simulink model "PMSM_ClosedLoop_s32k144"  (Simulink 9.0)
settings: Solver=FixedStepDiscrete  StartTime=0.0  StopTime=10  RelTol=1e-3  EnableMultiTasking=on
model workspace (MAT data in the model file):
  C_LST = 0.0001
  FORCE_MODE_SPEED = 20
  IDC_OVERCURRENT = 5
  IQ_REF_MAX = 2.3
  IQ_REF_TRACKING = 2
  I_MAX = 31.25
  Nmax = 10000
  PP = 2
  PhA_Offset = 16.025
  PhB_Offset = 16.04
  SPEED_DOWN_INC = 5
  SPEED_LOOP_CNTR = 10
  SPEED_UP_INC = 5
  S_LST = 0.001
  TRACKING_MODE_SPEED = 40
  VDC_OVERVOLTAGE = 18
  VDC_UNDERVOLTAGE = 8
InitFcn:
  | mbd_s32k_consistency_checks(bdroot(gcs));
undefined symbols (not defined in the file): External, LQFP, One, Shot, TRGMUX_PDB_TRIG
libraries: mbd_s32k1xx_ec_toolbox x50, ammclib_bam_s32k14x x26, simulink x18, mbd_msd_ec_toolbox x5
(part 1 of 2)
Description:
  | Closed Loop Speed Control PMSM example for S32K144 and DevKit MotorGD.
  | This Simulink model is designed to work with Linix 45ZWN24-40 Motor and validate
  | that the motor can be based on FOC method.
  | 
  | FEATURES:
  | - Speed command is read via SW2 (CW direction) or SW3 (CCW direction)
  | - Motor starts by default in CW direction. Use SW3 to decrease speed and move CCW.
  |   Alternatively, use FreeMASTER pannel to control the speed and direction
  | - Measure the 3-phase sinusoidal currents with PWM-PDB-ADC synchronization
  | - Measure the DC bus voltage and current with PWM-PDB-ADC synchronization
  | - PI Speed, Flux and Torque Controllers
  | - Speed estimator based on HALL sensors
  | 
  | HW SETUP:
  | - Configure S32K144 board supply voltage: J107:2-3(over USB)
  | - Configure J9,J10 and J11 on MotorGD: 2-3 (mode BLDC)
  | - Rotate trimmer resistor R72 (placed Devkit-MotorGD) counter-clockwise at maximum
  | - Connect the motor phases to MotorGD J13 connector
  |   (i.e. Linix 45ZWN24-40: phA-white/phB-blue/phC-green)
  | - Connect the motor hall sensors to MotorGD JP1 connector
  |   (i.e. Linix 45ZWN24-40: Hall_A-white/Hall_B-blue/Hall_C-green)
  | - Power on the MotorGD via J7 connector with 12Vdc
  | - NOTE! Make sure the R168/R166 are placed and R167/R165 are removed.
  |             Required for speed estimator based on hall sensor
  | 
  | VALIDATION:
  | - After reset or power on, the Green LED shall be ON
  | - In case of a FAULT the Red LED will be ON
  | - The initial speed command is set to 500rpm and can be changed from Simulink Model Wrks
  | - Open FreeMASTER project and connect to the target.
  | - Start by pressing the SW2 or SW3 to command the motor to spin
  | - Press the SW2 or SW3 the modify the motor speed or use FreeMASTER UI panel
  | - Voltage and Current protections for Devkit MotorGD are enabled. If fault occurs the
  |   INVERTER is shut down and RED LED is ON
  | 
  | NOTE:
  | - In case of fault (RED LED is ON), the remove fault cause and press RESET button
  | 
  | Copyright (c) 2019 NXP
  | version 3.2.0
settings Model: SuppressorTable="22 serialization::archive 15 0 6 0 0 1 8 0 0 0 0 6 0 0 1 0 97 PMSM_ClosedLoop_s32k144/S32K144 EVB/IO Controls/Alignment/Repeating Sequence Stair/LimitedCounter 0 6 0 0 2 8 0 0 0 0 6 40 SimulinkFixedPoint:util:Overflowoccurred 0 0 0 6 0  0  0 0 0 0 8 20160608 0 0 0 15 23 17 0 1 41 Simulink:DataType:WarningOverFlowDetected 0 0 0  0  8 20160608 0 15 23 17 0 1"  Creator=NXP MBDT Team  LastModifiedBy=nxf40284  OrderedModelArguments=off
settings DataIOCC: ExternalInput=off  InitialState=off  LimitDataPoints=on  SaveOutput=off  SignalLogging=off  SaveTime=off
settings OptimizationCC: DefaultParameterBehavior=Inlined  UseFloatMulNetSlope=on  DefaultUnderspecifiedDataType=single  UseSpecifiedMinMax=on  EnhancedBackFolding=on  PassReuseOutputArgsAs=Individual arguments  ZeroExternalMemoryAtStartup=off  ZeroInternalMemoryAtStartup=off  NoFixptDivByZeroProtection=on  EfficientFloat2IntCast=on  LifeSpan=auto  OptimizeBlockOrder=speed  DifferentSizesBufferReuse=on
settings DebuggingCC: CheckSSInitialOutputMsg=off  SolverPrmCheckMsg=warning  InheritedTsInSrcMsg=none  MultiTaskDSMMsg=none  SingleTaskRateTransMsg=error  ParameterPrecisionLossMsg=none  ParameterTunabilityLossMsg=error  UnconnectedInputMsg=error  UnconnectedOutputMsg=error  UnconnectedLineMsg=error  AssertControl=DisableAll  AllowSymbolicDim=off  UnknownTsInhSupMsg=error  StateNameClashWarn=warning  SFSelfTransitionDiag=none
settings HardwareCC: ProdLargestAtomicInteger=Long  ProdLargestAtomicFloat=Double  ProdIntDivRoundTo=Zero  ProdEndianess=LittleEndian  ProdHWDeviceType=ARM Compatible->ARM Cortex
settings ModelReferenceCC: PropagateSignalLabelsOutOfModel=on
settings SFSimCC: MATLABDynamicMemAlloc=off
settings RTWCC: SystemTargetFile=mbd_s32k.tlc  MakeCommand=mbd_s32k_make_rtw COPY_MDLREF_INCLUDES=0  TemplateMakefile=mbd_s32k.tmf  Description=Model Based Design Toolbox S32K1xx Code Generation Target  IncludeHyperlinkInReport=on
settings CodeAppCC: ForceParamTrailComments=on  IgnoreCustomStorageClasses=off  MaxIdLength=64  OperatorAnnotations=on  SimulinkDataObjDesc=on  SFDataObjDesc=on  InsertBlockDesc=on  StateflowObjectComments=off  InternalIdentifier=Classic
settings STFCustomTargetCC: TargetLangStandard=C99 (ISO)  MultiwordLength=256  CombineOutputUpdateFcns=on  ERTCustomFileBanners=on  SupportContinuousTime=off  SupportNonInlinedSFcns=off  RemoveResetFunc=on  MATLABClassNameForMDSCustomization=Simulink.SoftwareTarget.ERTCustomization  GRTInterface=off  SystemTargetFile=mbd_s32k.tlc
settings ERTTargetCC: TargetLangStandard=C99 (ISO)  ParMdlRefBuildCompliant=off  CompOptLevelCompliant=off  ConcurrentExecutionCompliant=off  ModelStepFunctionPrototypeControlCompliant=off  CPPClassGenCompliant=off  UseToolchainInfoCompliant=off  InlinedParameterPlacement=NonHierarchical  ERTSrcFileBannerTemplate=mbd_ert_code_template.cgt  ERTHdrFileBannerTemplate=mbd_ert_code_template.cgt  ERTDataSrcFileTemplate=mbd_ert_code_template.cgt  ERTDataHdrFileTemplate=mbd_ert_code_template.cgt  ERTCustomFileTemplate=example_file_process.tlc

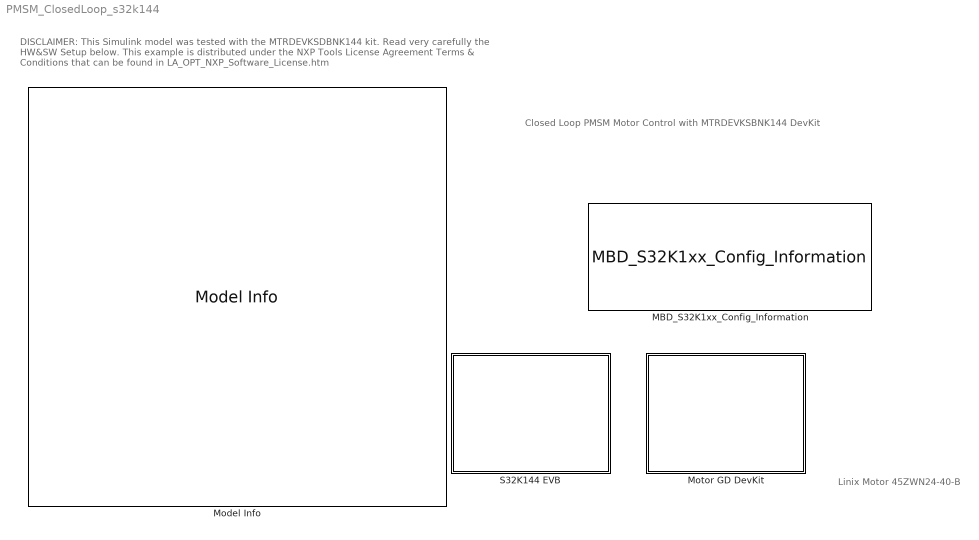
== system PMSM_ClosedLoop_s32k144 ==
  note: Linix Motor 45ZWN24-40-B
  note: Closed Loop PMSM Motor Control
      | with MTRDEVKSBNK144 DevKit
  note: DISCLAIMER: This Simulink model was tested with the MTRDEVKSDBNK144 kit. Read very carefully the HW&SW Setup below.
      | This example is distributed under the NXP Tools License Agreement Terms & Conditions that can be found in LA_OPT_NXP_Software_License.htm
  MBD_S32K1xx_Config_Information : mbd_s32k1xx_ec_toolbox/MBD_S32K1xx_Config_Information  mbdt_ver=0  disp_str=|  config_params=[]  mcu_target_name=S32K144  mcu_target_package=64-LQFP  mcu_target_sram_size=64KB  mcu_system_clock_freq=80  mcu_xtal_freq=External 8  mcu_steptick_timer=LPIT Channel 0  mcu_steptick_prio=15  ds_import_enable=on  target_compiler=GCC  target_memory=FLASH  gcc_target_compile_opts=-mcpu=cortex-m4 -mthumb -mfloat-abi=hard -mfpu=fpv4-sp-d16 -O1 -g -gstrict-dwarf  gcc_target_assemble_opts=-mcpu=cortex-m4 -mthumb -mfloat-abi=hard -mfpu=fpv4-sp-d16 -g  gcc_target_link_opts=-mcpu=cortex-m4 -mthumb -mfloat-abi=hard -mfpu=fpv4-sp-d16  gcc_target_default_lcf=on  gcc_target_user_lcf=S32K144_64_flash.ld  ghs_target_compile_opts=-cpu=cortexm4f -thumb -fpu=vfpv4_d16 -fsingle -Ogeneral -Wundef -Wimplicit-int -Wshadow -Wtrigraphs --no_commons --gnu_asm -gnu99 -gdwarf-2 -G  ghs_target_assemble_opts=-cpu=cortexm4f -fpu=vfpv4_d16  ghs_target_link_opts=-cpu=cortexm4f -thumb -fpu=vfpv4_d16  ghs_target_default_lcf=on  ghs_target_user_lcf=S32K144_64_flash.ld  iar_target_compile_opts=--cpu=Cortex-M4F --thumb --fpu=VFPv4_sp -Ol -e --debug --dlib_config normal  iar_target_assemble_opts=--cpu Cortex-M4F --thumb --fpu VFPv4_sp  iar_target_link_opts=--no_exceptions --vfe --inline  iar_target_default_lcf=on  iar_target_user_lcf=S32K144_64_flash.icf  pil_download_enable=off  rbl_download_enable=on  rbl_start_delay=5000  rbl_download_interface=OpenSDA  rbl_restart_request=off  rbl_com_port=Custom  rbl_com_port_custom=COM1  pil_download_rate=57600  pil_opensda_drive=Custom  pil_opensda_drive_custom=D  pil_uart_instance=1  pil_uart_rx=PTC6: [LPUART1_RX | Receive]  pil_uart_tx=PTC7: [LPUART1_TX | Transmit]  FTM_PWM_PcrCheckEnDis=on  FTM_Input_Edge_Inputs_PcrCheckEnDis=on  FTM_Dual_Edge_Inputs_PcrCheckEnDis=on  FTM_Quadrature_Inputs_PcrCheckEnDis=on  FTM_Hall_Sensor_Inputs_PcrCheckEnDis=on  LPTMR_PcrCheckEnDis=on  PIT_PcrCheckEnDis=on  RTC_PcrCheckEnDis=on  FlexCAN_PcrCheckEnDis=on  LIN_PcrCheckEnDis=on  FlexIO_PcrCheckEnDis=on  LPI2C_PcrCheckEnDis=on  LPSPI_PcrCheckEnDis=on  LPUART_PcrCheckEnDis=on  CMP_PcrCheckEnDis=on  GPIO_OutputPcrCheckEnDis=on  GPIO_InputPcrCheckEnDis=on  SBC_PcrCheckEnDis=on  AMMCLIB_PcrCheckEnDis=on  FM_PcrCheckEnDis=on  Profile_PcrCheckEnDis=on  ConfigParams_PcrCheckEnDis=on  ModelRef_PcrCheckEnDis=on  PDB0_PcrCheckEnDis=on  CSEc_PcrCheckEnDis=on  eDMA_PcrCheckEnDis=on  ADC_PcrCheckEnDis=on  WDOG_PcrCheckEnDis=on
      | Target : S32K144-64KB_SRAM
      | Package : 100-pin
      | System clock : 80 MHz
      | XTAL clock : External 8 MHz
      | Compiler : IAR
      | Target Type : FLASH
      | Download Code after build : off
      | Step Tick Interrupt Priority : 15
  Model Info : simulink/Model-Wide Utilities/Model Info  Frame=off  DisplayStringWithTags=|  HorizontalTextAlignment=Left  LeftAlignmentValue=0.02
      | Model Name: %<ModelName>
      | 
      | Description: %<Description>
  Motor GD DevKit : Subsystem
      mask Display: image('MotorGD.PNG');
  S32K144 EVB : Subsystem
      mask Display: image('S32K.PNG');

== system PMSM_ClosedLoop_s32k144/Motor GD DevKit ==

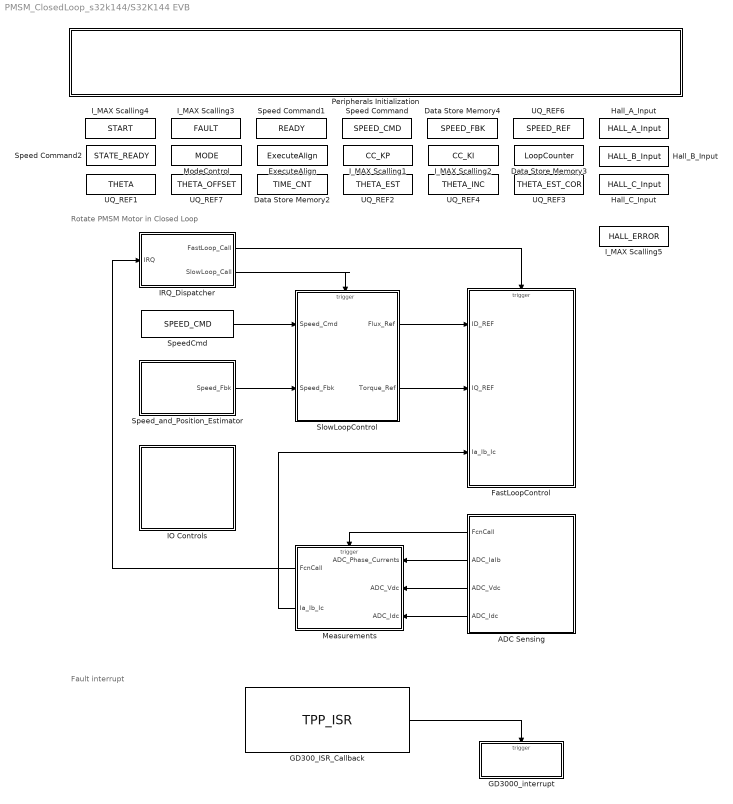
== system PMSM_ClosedLoop_s32k144/S32K144 EVB ==
  note: Rotate PMSM Motor in Closed Loop
  note: Fault interrupt
  ADC Sensing : Subsystem
  Data Store Memory2 : DataStoreMemory  DataStoreName=TIME_CNT  ReadBeforeWriteMsg=warning  WriteAfterWriteMsg=warning  WriteAfterReadMsg=warning  ShowAdditionalParam=off  OutDataTypeStr=uint32
  Data Store Memory3 : DataStoreMemory  DataStoreName=LoopCounter  ReadBeforeWriteMsg=warning  WriteAfterWriteMsg=warning  WriteAfterReadMsg=warning  ShowAdditionalParam=off  OutDataTypeStr=uint16
  Data Store Memory4 : DataStoreMemory  DataStoreName=SPEED_FBK  ReadBeforeWriteMsg=warning  WriteAfterWriteMsg=warning  WriteAfterReadMsg=warning  ShowAdditionalParam=off  OutDataTypeStr=single
      settings: RTWStateStorageClass=ExportedGlobal
  ExecuteAlign : DataStoreMemory  DataStoreName=ExecuteAlign  ReadBeforeWriteMsg=warning  WriteAfterWriteMsg=warning  WriteAfterReadMsg=warning  ShowAdditionalParam=off  OutDataTypeStr=boolean
      settings: RTWStateStorageClass=ExportedGlobal
  FastLoopControl : Subsystem
      settings: RTWSystemCode=Nonreusable function  RTWFcnNameOpts=Use subsystem name
  GD3000_interrupt : Subsystem  TreatAsAtomicUnit=on
  "GD300_ISR_Callback " : mbd_msd_ec_toolbox/TPP/TPP_ISR  tppInstance=0
  Hall_A_Input : DataStoreMemory  DataStoreName=HALL_A_Input  ReadBeforeWriteMsg=warning  WriteAfterWriteMsg=warning  WriteAfterReadMsg=warning  ShowAdditionalParam=off  OutDataTypeStr=boolean
  Hall_B_Input : DataStoreMemory  DataStoreName=HALL_B_Input  ReadBeforeWriteMsg=warning  WriteAfterWriteMsg=warning  WriteAfterReadMsg=warning  ShowAdditionalParam=off  OutDataTypeStr=boolean
  Hall_C_Input : DataStoreMemory  DataStoreName=HALL_C_Input  ReadBeforeWriteMsg=warning  WriteAfterWriteMsg=warning  WriteAfterReadMsg=warning  ShowAdditionalParam=off  OutDataTypeStr=boolean
  IO Controls : Subsystem
  IRQ_Dispatcher : Subsystem
      settings: MinAlgLoopOccurrences=on
  I_MAX Scalling1 : DataStoreMemory  DataStoreName=CC_KP  ReadBeforeWriteMsg=warning  WriteAfterWriteMsg=warning  WriteAfterReadMsg=warning  InitialValue=0.2  ShowAdditionalParam=off  OutDataTypeStr=single
  I_MAX Scalling2 : DataStoreMemory  DataStoreName=CC_KI  ReadBeforeWriteMsg=warning  WriteAfterWriteMsg=warning  WriteAfterReadMsg=warning  InitialValue=0.25  ShowAdditionalParam=off  OutDataTypeStr=single
  I_MAX Scalling3 : DataStoreMemory  DataStoreName=FAULT  ReadBeforeWriteMsg=warning  WriteAfterWriteMsg=warning  WriteAfterReadMsg=warning  ShowAdditionalParam=off  OutDataTypeStr=boolean
  I_MAX Scalling4 : DataStoreMemory  DataStoreName=START  ReadBeforeWriteMsg=warning  WriteAfterWriteMsg=warning  WriteAfterReadMsg=warning  ShowAdditionalParam=off  OutDataTypeStr=boolean
  I_MAX Scalling5 : DataStoreMemory  DataStoreName=HALL_ERROR  ReadBeforeWriteMsg=warning  WriteAfterWriteMsg=warning  WriteAfterReadMsg=warning  ShowAdditionalParam=off  OutDataTypeStr=uint8
  Measurements : Subsystem  TreatAsAtomicUnit=on
  ModeControl : DataStoreMemory  DataStoreName=MODE  ReadBeforeWriteMsg=warning  WriteAfterWriteMsg=warning  WriteAfterReadMsg=warning  ShowAdditionalParam=off  OutMin=0  OutMax=2  OutDataTypeStr=uint16
      settings: RTWStateStorageClass=ExportedGlobal
  Peripherals Initialization : Subsystem  Priority=1
  SlowLoopControl : Subsystem
      settings: PropExecContextOutsideSubsystem=on  RTWSystemCode=Nonreusable function  RTWFcnNameOpts=Use subsystem name
  Speed Command : DataStoreMemory  DataStoreName=SPEED_CMD  ReadBeforeWriteMsg=warning  WriteAfterWriteMsg=warning  WriteAfterReadMsg=warning  InitialValue=52.35  ShowAdditionalParam=off  OutMin=0  OutMax=209.4  OutDataTypeStr=single
  Speed Command1 : DataStoreMemory  DataStoreName=READY  ReadBeforeWriteMsg=warning  WriteAfterWriteMsg=warning  WriteAfterReadMsg=warning  ShowAdditionalParam=off  OutMin=0  OutMax=1  OutDataTypeStr=boolean
  Speed Command2 : DataStoreMemory  DataStoreName=STATE_READY  ReadBeforeWriteMsg=warning  WriteAfterWriteMsg=warning  WriteAfterReadMsg=warning  ShowAdditionalParam=off  OutMin=0  OutMax=1  OutDataTypeStr=boolean
  SpeedCmd : DataStoreRead  DataStoreName=SPEED_CMD
  Speed_and_Position_Estimator : Subsystem  TreatAsAtomicUnit=on
      settings: RTWFcnNameOpts=Use subsystem name
  UQ_REF1 : DataStoreMemory  DataStoreName=THETA  ReadBeforeWriteMsg=warning  WriteAfterWriteMsg=warning  WriteAfterReadMsg=warning  ShowAdditionalParam=off  OutDataTypeStr=single
  UQ_REF2 : DataStoreMemory  DataStoreName=THETA_EST  ReadBeforeWriteMsg=warning  WriteAfterWriteMsg=warning  WriteAfterReadMsg=warning  ShowAdditionalParam=off  OutDataTypeStr=single
  UQ_REF3 : DataStoreMemory  DataStoreName=THETA_EST_COR  ReadBeforeWriteMsg=warning  WriteAfterWriteMsg=warning  WriteAfterReadMsg=warning  ShowAdditionalParam=off  OutDataTypeStr=single
  UQ_REF4 : DataStoreMemory  DataStoreName=THETA_INC  ReadBeforeWriteMsg=warning  WriteAfterWriteMsg=warning  WriteAfterReadMsg=warning  ShowAdditionalParam=off  OutDataTypeStr=single
  UQ_REF6 : DataStoreMemory  DataStoreName=SPEED_REF  ReadBeforeWriteMsg=warning  WriteAfterWriteMsg=warning  WriteAfterReadMsg=warning  ShowAdditionalParam=off  OutDataTypeStr=single
  UQ_REF7 : DataStoreMemory  DataStoreName=THETA_OFFSET  ReadBeforeWriteMsg=warning  WriteAfterWriteMsg=warning  WriteAfterReadMsg=warning  ShowAdditionalParam=off  OutDataTypeStr=single
  wires:
  Measurements/2(Ia_Ib_Ic) -> FastLoopControl/3(Ia_Ib_Ic)
  ADC Sensing/2(ADC_IaIb) -> Measurements/1(ADC_Phase_Currents)
  SlowLoopControl/2(Torque_Ref) -> FastLoopControl/2(IQ_REF)
  Measurements/1(FcnCall) -> IRQ_Dispatcher/1(IRQ)
  ADC Sensing/1(FcnCall) -> Measurements/Trigger
  ADC Sensing/3(ADC_Vdc) -> Measurements/2(ADC_Vdc)
  SlowLoopControl/1(Flux_Ref) -> FastLoopControl/1(ID_REF)
  IRQ_Dispatcher/2(SlowLoop_Call) -> SlowLoopControl/Trigger
  ADC Sensing/4(ADC_Idc) -> Measurements/3(ADC_Idc)
  IRQ_Dispatcher/1(FastLoop_Call) -> FastLoopControl/Trigger
  SpeedCmd/1 -> SlowLoopControl/1(Speed_Cmd)
  Speed_and_Position_Estimator/1(Speed_Fbk) -> SlowLoopControl/2(Speed_Fbk)
  "GD300_ISR_Callback "/1 -> GD3000_interrupt/Trigger

== system PMSM_ClosedLoop_s32k144/S32K144 EVB/ADC Sensing ==
  ADC1_IRQHandler : Subsystem  TreatAsAtomicUnit=on
  ADC1_ISR : mbd_s32k1xx_ec_toolbox/Motor Control Blocks/ADC Blocks/ADC_ISR  instance=1  pri=1  sc1n=C
  PDB1_IRQHandler : Subsystem  TreatAsAtomicUnit=on
  PDB1_ISR : mbd_s32k1xx_ec_toolbox/Motor Control Blocks/PDB Blocks/PDB_ISR  Priority=8  pdbModule=1  prioInterrupt=2  regScPdbie=on  regScPdbeie=off  regIdlyIdly=4999
  Terminator{,1..2,6} (4 alike) : Terminator
  FcnCall : Outport
  ADC_IaIb : Outport  Port=2
  ADC_Vdc : Outport  Port=3
  ADC_Idc : Outport  Port=4
  wires:
  PDB1_ISR/2 -> Terminator1/1
  PDB1_ISR/3 -> Terminator2/1
  PDB1_ISR/4 -> Terminator/1
  PDB1_ISR/1 -> PDB1_IRQHandler/Trigger
  ADC1_IRQHandler/3(ADC_Vdc) -> ADC_Vdc/1
  ADC1_IRQHandler/2(ADC_Phase_Currents) -> ADC_IaIb/1
  ADC1_IRQHandler/4(ADC_Idc) -> ADC_Idc/1
  ADC1_IRQHandler/1(FcnCall) -> FcnCall/1
  ADC1_ISR/1 -> ADC1_IRQHandler/Trigger
  ADC1_ISR/2 -> ADC1_IRQHandler/1(ADC_IB)
  ADC1_ISR/3 -> Terminator6/1

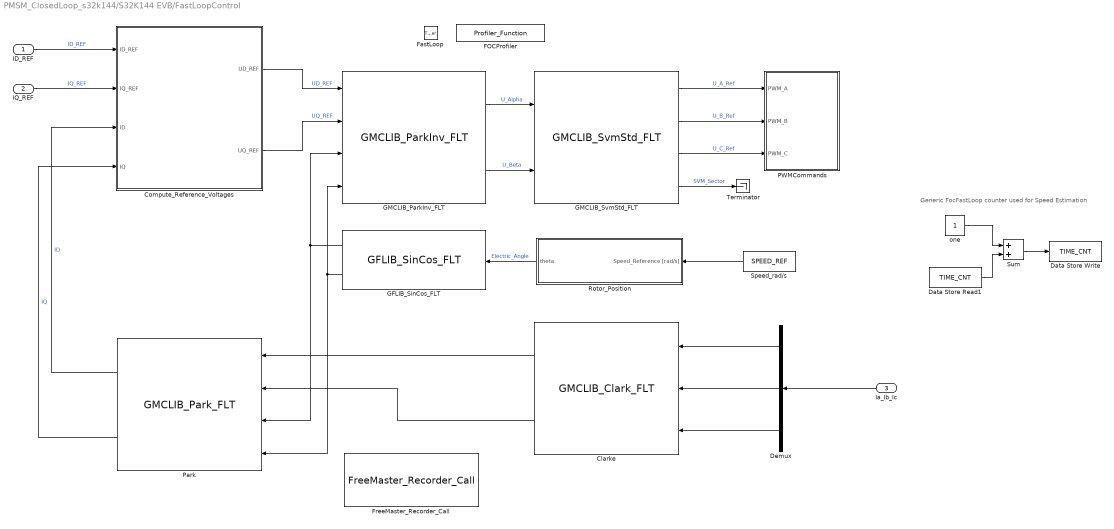
== system PMSM_ClosedLoop_s32k144/S32K144 EVB/FastLoopControl ==
  note: Generic FocFastLoop counter used for Speed Estimation
  ID_REF : Inport
  IQ_REF : Inport  Port=2
  Ia_Ib_Ic : Inport  Port=3
  FastLoop : TriggerPort  TriggerType=function-call  VariantControl=(inherit)
  Clarke : ammclib_bam_s32k14x/GMCLIB/bam_flt/GMCLIB_Clark_FLT
  Compute_Reference_Voltages : Subsystem
  Data Store Read1 : DataStoreRead  DataStoreName=TIME_CNT
  Data Store Write : DataStoreWrite  DataStoreName=TIME_CNT
  Demux : Demux  Outputs=3
  FOCProfiler : mbd_s32k1xx_ec_toolbox/Utility Blocks/Profiler_Function  profile_indx=2
  FreeMaster_Recorder_Call : mbd_s32k1xx_ec_toolbox/Utility Blocks/FreeMaster_Recorder_Call
  GFLIB_SinCos_FLT : ammclib_bam_s32k14x/GFLIB/bam_flt/GFLIB_SinCos_FLT
  GMCLIB_ParkInv_FLT : ammclib_bam_s32k14x/GMCLIB/bam_flt/GMCLIB_ParkInv_FLT
  GMCLIB_SvmStd_FLT : ammclib_bam_s32k14x/GMCLIB/bam_flt/GMCLIB_SvmStd_FLT
  PWMCommands : Subsystem
  Park : ammclib_bam_s32k14x/GMCLIB/bam_flt/GMCLIB_Park_FLT
  Rotor_Position : Subsystem
  Speed_rad/s : DataStoreRead  DataStoreName=SPEED_REF
  Sum : Sum
  Terminator : Terminator
  one : Constant  OutDataTypeStr=uint32
  wires:
  GFLIB_SinCos_FLT/2 -> Park/4, GMCLIB_ParkInv_FLT/4
  GMCLIB_ParkInv_FLT/1 -> GMCLIB_SvmStd_FLT/1  "U_Alpha"
  GMCLIB_ParkInv_FLT/2 -> GMCLIB_SvmStd_FLT/2  "U_Beta"
  GFLIB_SinCos_FLT/1 -> Park/3, GMCLIB_ParkInv_FLT/3
  GMCLIB_SvmStd_FLT/2 -> PWMCommands/2(PWM_B)  "U_B_Ref"
  GMCLIB_SvmStd_FLT/3 -> PWMCommands/3(PWM_C)  "U_C_Ref"
  GMCLIB_SvmStd_FLT/4 -> Terminator/1  "SVM_Sector"
  GMCLIB_SvmStd_FLT/1 -> PWMCommands/1(PWM_A)  "U_A_Ref"
  Compute_Reference_Voltages/1(UD_REF) -> GMCLIB_ParkInv_FLT/1  "UD_REF"
  Compute_Reference_Voltages/2(UQ_REF) -> GMCLIB_ParkInv_FLT/2  "UQ_REF"
  Rotor_Position/1(theta) -> GFLIB_SinCos_FLT/1  "Electric_Angle"
  Park/1 -> Compute_Reference_Voltages/3(ID)  "ID"
  IQ_REF/1 -> Compute_Reference_Voltages/2(IQ_REF)  "IQ_REF"
  Park/2 -> Compute_Reference_Voltages/4(IQ)  "IQ"
  ID_REF/1 -> Compute_Reference_Voltages/1(ID_REF)  "ID_REF"
  Demux/2 -> Clarke/2
  Demux/3 -> Clarke/3
  Ia_Ib_Ic/1 -> Demux/1
  Clarke/1 -> Park/1
  Clarke/2 -> Park/2
  Demux/1 -> Clarke/1
  one/1 -> Sum/1
  Data Store Read1/1 -> Sum/2
  Speed_rad/s/1 -> Rotor_Position/1(Speed_Reference [rad/s])
  Sum/1 -> Data Store Write/1

== system PMSM_ClosedLoop_s32k144/S32K144 EVB/GD3000_interrupt ==
  function : TriggerPort  TriggerType=function-call  VariantControl=Variant
  FAULT_write : DataStoreWrite  DataStoreName=FAULT
  FTM_PWM_Disable_Enable : mbd_s32k1xx_ec_toolbox/Motor Control Blocks/FTM Blocks/FTM_PWM_Disable_Enable  ftmModule=3  action=Disable
  NOK : Constant  OutDataTypeStr=boolean
  TPP_Functional_Mode : mbd_msd_ec_toolbox/TPP/TPP_Functional_Mode  tppInstance=0  action=Sleep
  wires:
  NOK/1 -> FAULT_write/1

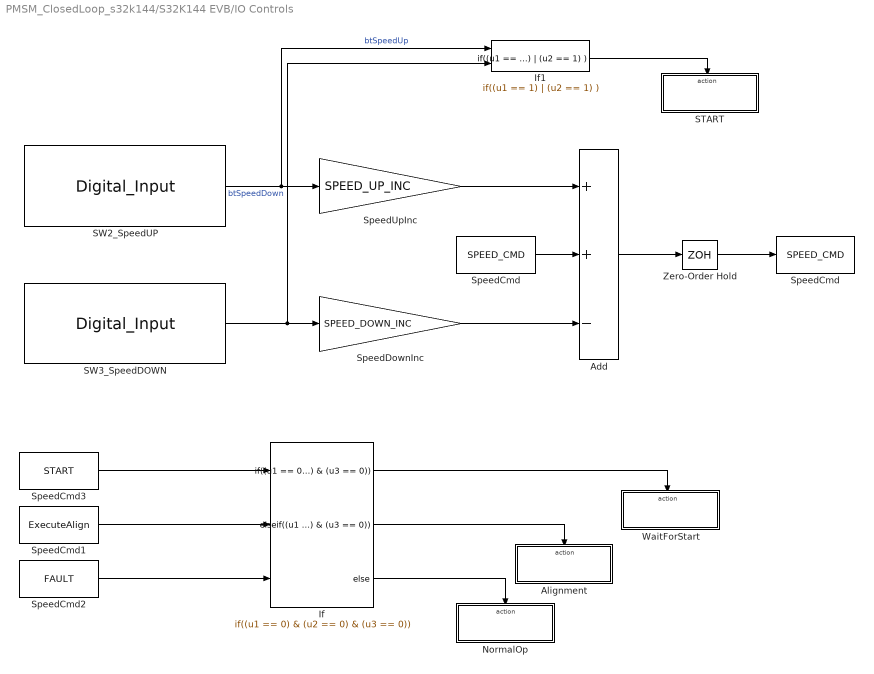
== system PMSM_ClosedLoop_s32k144/S32K144 EVB/IO Controls ==
  Add : Sum  Inputs=++-
  Alignment : Subsystem  TreatAsAtomicUnit=on
  If : If  NumInputs=3  IfExpression=(u1 == 0) & (u2 == 0) & (u3 == 0)  ElseIfExpressions=(u1 == 1) & (u2 ~= 0) & (u3 == 0)
  If1 : If  NumInputs=2  IfExpression=(u1 == 1) | (u2 == 1)  ShowElse=off
  NormalOp : Subsystem  TreatAsAtomicUnit=on
  START : Subsystem  TreatAsAtomicUnit=on
  SW2_SpeedUP : mbd_s32k1xx_ec_toolbox/GPIO Blocks/Digital_Input  gpio_pin=PTC12: [PTC12 | Port C I/O]  pull_resistor=None  passive_filter=off
  SW3_SpeedDOWN : mbd_s32k1xx_ec_toolbox/GPIO Blocks/Digital_Input  gpio_pin=PTC13: [PTC13 | Port C I/O]  pull_resistor=None  passive_filter=off
  SpeedCmd : DataStoreRead  DataStoreName=SPEED_CMD
  "SpeedCmd " : DataStoreWrite  DataStoreName=SPEED_CMD
  SpeedCmd1 : DataStoreRead  DataStoreName=ExecuteAlign
  SpeedCmd2 : DataStoreRead  DataStoreName=FAULT
  SpeedCmd3 : DataStoreRead  DataStoreName=START
  SpeedDownInc : Gain  Gain=SPEED_DOWN_INC  OutDataTypeStr=single
  SpeedUpInc : Gain  Gain=SPEED_UP_INC  OutDataTypeStr=single
  WaitForStart : Subsystem  TreatAsAtomicUnit=on
  Zero-Order Hold : ZeroOrderHold  SampleTime=0.25
  wires:
  Add/1 -> Zero-Order Hold/1
  SW3_SpeedDOWN/1 -> If1/2, SpeedDownInc/1  "btSpeedDown"
  SW2_SpeedUP/1 -> If1/1, SpeedUpInc/1  "btSpeedUp"
  SpeedCmd/1 -> Add/2
  SpeedUpInc/1 -> Add/1
  SpeedDownInc/1 -> Add/3
  Zero-Order Hold/1 -> "SpeedCmd "/1
  If1/1 -> START/Action
  SpeedCmd2/1 -> If/3
  SpeedCmd3/1 -> If/1
  If/1 -> WaitForStart/Action
  If/3 -> NormalOp/Action
  SpeedCmd1/1 -> If/2
  If/2 -> Alignment/Action

== system PMSM_ClosedLoop_s32k144/S32K144 EVB/IRQ_Dispatcher ==
  IRQ : Inport
  " " : DataStoreRead  DataStoreName=READY
  "  " : DataStoreRead  DataStoreName=START
  Generate_Triggers : Subsystem  TreatAsAtomicUnit=on
  Generate_Triggers_on_Startup : If  NumInputs=2  IfExpression=(u1 == 0) & (u2 == 1)  ShowElse=off
  Mux1 : Mux  Inputs=2
  Trigger_FastLoop_Call : Subsystem  TreatAsAtomicUnit=on
  FastLoop_Call : Outport
  SlowLoop_Call : Outport  Port=2
  wires:
  " "/1 -> Generate_Triggers_on_Startup/1
  Generate_Triggers_on_Startup/1 -> Trigger_FastLoop_Call/Action
  Trigger_FastLoop_Call/1(Call) -> Mux1/1
  Mux1/1 -> FastLoop_Call/1
  IRQ/1 -> Generate_Triggers/Trigger
  Generate_Triggers/1(FastLoop_Call) -> Mux1/2
  Generate_Triggers/2(SlowLoop_Call) -> SlowLoop_Call/1
  "  "/1 -> Generate_Triggers_on_Startup/2

== system PMSM_ClosedLoop_s32k144/S32K144 EVB/Measurements ==
  ADC_Phase_Currents : Inport
  ADC_Vdc : Inport  Port=2
  ADC_Idc : Inport  Port=3
  function : TriggerPort  TriggerType=function-call  VariantControl=(inherit)
  FaultDetection : Subsystem  TreatAsAtomicUnit=on
  Function-Call Generator : simulink/Ports & Subsystems/Function-Call Generator  Priority=4  sample_time=-1  numberOfIterations=1
  Get3PhCurrent : Subsystem  Priority=1  TreatAsAtomicUnit=on
  GetIdcCurrent : Subsystem  Priority=3  TreatAsAtomicUnit=on
      settings: RTWFcnNameOpts=Use subsystem name
  GetVdcVoltage : Subsystem  Priority=2  TreatAsAtomicUnit=on
      settings: RTWFcnNameOpts=Use subsystem name
  FcnCall : Outport
  Ia_Ib_Ic : Outport  Port=2
  wires:
  ADC_Vdc/1 -> GetVdcVoltage/1(ADC_Vdc)
  GetIdcCurrent/1(Idc) -> FaultDetection/2(Idc)
  GetVdcVoltage/1(Vdc) -> FaultDetection/1(Vdc)
  ADC_Phase_Currents/1 -> Get3PhCurrent/1(ADC_Phase_Currents)
  ADC_Idc/1 -> GetIdcCurrent/1(ADC_Idc)
  Get3PhCurrent/1(Ia_Ib_Ic) -> Ia_Ib_Ic/1
  Function-Call Generator/1 -> FcnCall/1

== system PMSM_ClosedLoop_s32k144/S32K144 EVB/Peripherals Initialization ==
  ADC0_Init : mbd_s32k1xx_ec_toolbox/Motor Control Blocks/ADC Blocks/ADC_Config  Priority=3  instance=0  mode=12-bit conversion  smplts=2  adiclk=alternate clock 1  adiv=input clock  show_adv_opts=on  pretrgsel=PDB pre-trigger  swpretrg=Disabled  adtrg=hardware  trgsel=PDB output  refsel=Vrefh and Vrefl  supply_monitoring=off  acfe=off  acfgt=off  acren=off  cv1=0  cv2=0  adco=off  avge=off  avgs=4 samples
  ADC1_IRQ : mbd_s32k1xx_ec_toolbox/Motor Control Blocks/ADC Blocks/ADC_Start  Priority=5  instance=1  adc_r=C  adc_chan=PTB16: [ADC1_SE15 | ADC Single Ended Input]  aien=on  mcuTargetUpdate=on
  ADC1_Init : mbd_s32k1xx_ec_toolbox/Motor Control Blocks/ADC Blocks/ADC_Config  Priority=4  instance=1  mode=12-bit conversion  smplts=2  adiclk=alternate clock 1  adiv=input clock  show_adv_opts=on  pretrgsel=PDB pre-trigger  swpretrg=Disabled  adtrg=hardware  trgsel=PDB output  refsel=Vrefh and Vrefl  supply_monitoring=off  acfe=off  acfgt=off  acren=off  cv1=0  cv2=0  adco=off  avge=off  avgs=4 samples
  ADC_Interleave : mbd_s32k1xx_ec_toolbox/Motor Control Blocks/ADC Blocks/ADC_Interleave  adcInterleavePins=PTB1 to ADC0_SE5 and ADC1_SE15  adcInterleaveInit=on
  FreeMaster_Config : mbd_s32k1xx_ec_toolbox/Utility Blocks/FreeMaster_Config  interface=LPUART1  baudrate=115200  rxd=PTC6: [LPUART1_RX | Receive]  txd=PTC7: [LPUART1_TX | Transmit]  mode=Short Interrupt  isr_prio=10  show_adv_opts=on  use_scope=on  max_scope_vars=8  use_recorder=on  max_rec_vars=8  rec_buff_size=8192  rec_timebase=100 microseconds  comm_buffer_size_auto=on  comm_buffer_size=255  comm_rqueue_size_default=on  comm_rqueue_size=32
  GD3000_Config : mbd_msd_ec_toolbox/TPP/TPP_Config  Priority=1  tppInstance=0  desatMode=on  fullonMode=off  lockMode=off  overtempEvent=on  phaseEvent=off  desatEvent=off  framingEvent=on  vlsEvent=on  writeErrEvent=on  overcurrentEvent=on  resetEvent=on  mcuTppIntEn=off  prioInt=15  tppDeadtime=500  initTppNow=on  tppSpiInst=Please add SPI block to workspace  tppPwmModule=Please add FTM block to workspace  tppPair0_1=on  tppPair2_3=on  tppPair4_5=on  tppPair6_7=off  tppFirstChHS=on  tppEn1Pin=PTA2: [PTA2 | Port A I/O]  tppEn2Pin=PTA2: [PTA2 | Port A I/O]  tppRstPin=PTA3: [PTA3 | Port A I/O]  tppCsPin=PTB5: [PTB5 | Port B I/O]  tppIntPin=PTE10: [PTE10 | Port E I/O]
  "LPSPI_Config " : mbd_s32k1xx_ec_toolbox/Communication Blocks/SPI Blocks/LPSPI_Config   InstanceNumber=0  Role=Master  BaudRate=1000000  ShowAdvanced=on  sin=PTB3: [LPSPI0_SIN | LPSPI Serial Data Input]  sout=PTB4: [LPSPI0_SOUT | LPSPI Serial Data Output]  sck=PTB2: [LPSPI0_SCK | LPSPI Serial Clock I/O]  pcs0=None  pcs1=PTB5: [LPSPI0_PCS1 | Peripheral Chip Select 1]  pcs2=None  pcs3=None  CPHA=1  CPOL=0  BitOrder=MSB first  TransferSize=8  WhichPCS=1  PCSPol=ActiveLow  ContinuousTransfer=off
  PDB0_Init : mbd_s32k1xx_ec_toolbox/Motor Control Blocks/PDB Blocks/PDB_Config  Priority=1  pdbModule=0  regScCont=One-Shot  regScTrgsel=External (TRGMUX_PDB_TRIG)  trgMuxSel=FTM3 Initialize Trigger  trgMuxSelPin=PTB5: [TRGMUX_IN0 | Trigger Mux Input]  regModModulus=5000  regScPrescaler=1  regScMult=1  regPoenPoen0=off  regPo0DlyDly1=0  regPo0DlyDly2=0  enable_pdb_init=off  show_adv_opts=on  regCh0C1En0=on  regCh0C1En1=off  regCh0C1En2=off  regCh0C1En3=off  regCh0C1En4=off  regCh0C1En5=off  regCh0C1En6=off  regCh0C1En7=off  regCh0C1Bb0=off  regCh0C1Bb1=off  regCh0C1Bb2=off  regCh0C1Bb3=off  regCh0C1Bb4=off  regCh0C1Bb5=off  regCh0C1Bb6=off  regCh0C1Bb7=off  regCh0C1Tos0=Pre-trigger is in delay mode  regCh0C1Tos1=Pre-trigger is in delay mode  regCh0C1Tos2=Pre-trigger is in delay mode  regCh0C1Tos3=Pre-trigger is in delay mode  regCh0C1Tos4=Pre-trigger is in delay mode  regCh0C1Tos5=Pre-trigger is in delay mode  regCh0C1Tos6=Pre-trigger is in delay mode  regCh0C1Tos7=Pre-trigger is in delay mode  regCh0DlyDly0=2000  regCh0DlyDly1=0  regCh0DlyDly2=0  regCh0DlyDly3=0  regCh0DlyDly4=0  regCh0DlyDly5=0  regCh0DlyDly6=0  regCh0DlyDly7=0  regCh1C1En0=off  regCh1C1En1=off  regCh1C1En2=off  regCh1C1En3=off  regCh1C1En4=off  regCh1C1En5=off  regCh1C1En6=off  regCh1C1En7=off  regCh1C1Bb0=off  regCh1C1Bb1=off  regCh1C1Bb2=off  regCh1C1Bb3=off  regCh1C1Bb4=off  regCh1C1Bb5=off  regCh1C1Bb6=off  regCh1C1Bb7=off  regCh1C1Tos0=Pre-trigger is in delay mode  regCh1C1Tos1=Pre-trigger is in delay mode  regCh1C1Tos2=Pre-trigger is in delay mode  regCh1C1Tos3=Pre-trigger is in delay mode  regCh1C1Tos4=Pre-trigger is in delay mode  regCh1C1Tos5=Pre-trigger is in delay mode  regCh1C1Tos6=Pre-trigger is in delay mode  regCh1C1Tos7=Pre-trigger is in delay mode  regCh1DlyDly0=0  regCh1DlyDly1=0  regCh1DlyDly2=0  regCh1DlyDly3=0  regCh1DlyDly4=0  regCh1DlyDly5=0  regCh1DlyDly6=0  regCh1DlyDly7=0
  PDB1_Init : mbd_s32k1xx_ec_toolbox/Motor Control Blocks/PDB Blocks/PDB_Config  Priority=2  pdbModule=1  regScCont=One-Shot  regScTrgsel=External (TRGMUX_PDB_TRIG)  trgMuxSel=FTM3 Initialize Trigger  trgMuxSelPin=PTB5: [TRGMUX_IN0 | Trigger Mux Input]  regModModulus=5000  regScPrescaler=1  regScMult=1  regPoenPoen0=off  regPo0DlyDly1=0  regPo0DlyDly2=0  enable_pdb_init=off  show_adv_opts=on  regCh0C1En0=on  regCh0C1En1=on  regCh0C1En2=on  regCh0C1En3=off  regCh0C1En4=off  regCh0C1En5=off  regCh0C1En6=off  regCh0C1En7=off  regCh0C1Bb0=off  regCh0C1Bb1=off  regCh0C1Bb2=off  regCh0C1Bb3=off  regCh0C1Bb4=off  regCh0C1Bb5=off  regCh0C1Bb6=off  regCh0C1Bb7=off  regCh0C1Tos0=Pre-trigger is in delay mode  regCh0C1Tos1=Pre-trigger is in delay mode  regCh0C1Tos2=Pre-trigger is in delay mode  regCh0C1Tos3=Pre-trigger is in delay mode  regCh0C1Tos4=Pre-trigger is in delay mode  regCh0C1Tos5=Pre-trigger is in delay mode  regCh0C1Tos6=Pre-trigger is in delay mode  regCh0C1Tos7=Pre-trigger is in delay mode  regCh0DlyDly0=0  regCh0DlyDly1=1000  regCh0DlyDly2=2000  regCh0DlyDly3=0  regCh0DlyDly4=0  regCh0DlyDly5=0  regCh0DlyDly6=0  regCh0DlyDly7=0  regCh1C1En0=off  regCh1C1En1=off  regCh1C1En2=off  regCh1C1En3=off  regCh1C1En4=off  regCh1C1En5=off  regCh1C1En6=off  regCh1C1En7=off  regCh1C1Bb0=off  regCh1C1Bb1=off  regCh1C1Bb2=off  regCh1C1Bb3=off  regCh1C1Bb4=off  regCh1C1Bb5=off  regCh1C1Bb6=off  regCh1C1Bb7=off  regCh1C1Tos0=Pre-trigger is in delay mode  regCh1C1Tos1=Pre-trigger is in delay mode  regCh1C1Tos2=Pre-trigger is in delay mode  regCh1C1Tos3=Pre-trigger is in delay mode  regCh1C1Tos4=Pre-trigger is in delay mode  regCh1C1Tos5=Pre-trigger is in delay mode  regCh1C1Tos6=Pre-trigger is in delay mode  regCh1C1Tos7=Pre-trigger is in delay mode  regCh1DlyDly0=0  regCh1DlyDly1=0  regCh1DlyDly2=0  regCh1DlyDly3=0  regCh1DlyDly4=0  regCh1DlyDly5=0  regCh1DlyDly6=0  regCh1DlyDly7=0

== system PMSM_ClosedLoop_s32k144/S32K144 EVB/SlowLoopControl ==
  Speed_Cmd : Inport
  Speed_Fbk : Inport  Port=2
  SlowLoop : TriggerPort  TriggerType=function-call  VariantControl=(inherit)
  Alignment_vs_NormalOp_Sequence : Subsystem  TreatAsAtomicUnit=on
      settings: RTWSystemCode=Nonreusable function  RTWFcnNameOpts=Use subsystem name
  Compute_Positioning_Mode : Subsystem  TreatAsAtomicUnit=on
      settings: RTWSystemCode=Nonreusable function  RTWFcnNameOpts=Use subsystem name
  D_axis_flux : Constant  Value=0  OutDataTypeStr=single  SampleTime=-1
  Generate_Speed_Reference : Subsystem  TreatAsAtomicUnit=on
      settings: RTWSystemCode=Nonreusable function  RTWFcnNameOpts=Use subsystem name
  SlowLoopProfiler : mbd_s32k1xx_ec_toolbox/Utility Blocks/Profiler_Function  profile_indx=1
  Speed_Controller : Subsystem  TreatAsAtomicUnit=on
      settings: RTWSystemCode=Nonreusable function  RTWFcnNameOpts=Use subsystem name
  Update_Theta_Offset : Subsystem
  Flux_Ref : Outport
  Torque_Ref : Outport  Port=2
  wires:
  Speed_Controller/1(Torque_Cmd) -> Alignment_vs_NormalOp_Sequence/1(Torque_Cmd)
  D_axis_flux/1 -> Alignment_vs_NormalOp_Sequence/2(Flux_Cmd)
  Speed_Cmd/1 -> Generate_Speed_Reference/1(Speed_Cmd)
  Generate_Speed_Reference/1(Speed_Ref) -> Update_Theta_Offset/1(Speed_Ref), Compute_Positioning_Mode/1(Speed_Ref), Speed_Controller/1(Speed_Ref)
  Alignment_vs_NormalOp_Sequence/1(Torque_Ref) -> Torque_Ref/1
  Speed_Fbk/1 -> Speed_Controller/2(Speed_Fbk)
  Alignment_vs_NormalOp_Sequence/2(Flux_Ref) -> Flux_Ref/1

== system PMSM_ClosedLoop_s32k144/S32K144 EVB/Speed_and_Position_Estimator ==
  note: Estimate the motor speed based on HALL transitions and FocFastLoop counter
  Estimate_Position : Subsystem
  HALL_A : mbd_s32k1xx_ec_toolbox/GPIO Blocks/Digital_Input_ISR  gpio_pin=PTD11: [PTD11 | Port D I/O]  irqc=on either-edge  prio=5
  HALL_B : mbd_s32k1xx_ec_toolbox/GPIO Blocks/Digital_Input_ISR  gpio_pin=PTD10: [PTD10 | Port D I/O]  irqc=on either-edge  prio=5
  HALL_C : mbd_s32k1xx_ec_toolbox/GPIO Blocks/Digital_Input_ISR  gpio_pin=PTA1: [PTA1 | Port A I/O]  irqc=on either-edge  prio=5
  Mux : Mux  Inputs=3
  SpeedEstimatorProfiler : mbd_s32k1xx_ec_toolbox/Utility Blocks/Profiler_Function  profile_indx=3
  Update_HALL_A : Subsystem
  Update_HALL_B : Subsystem
  Update_HALL_C_Estimate_Speed : Subsystem
  Speed_Fbk : Outport
  wires:
  Mux/1 -> Estimate_Position/Trigger
  Update_HALL_A/1(Call) -> Mux/1
  HALL_B/1 -> Update_HALL_B/Trigger
  HALL_A/1 -> Update_HALL_A/Trigger
  Update_HALL_B/1(Call) -> Mux/2
  Update_HALL_C_Estimate_Speed/1(Call) -> Mux/3
  HALL_C/1 -> Update_HALL_C_Estimate_Speed/Trigger
  Update_HALL_C_Estimate_Speed/2(Speed_Fbk) -> Speed_Fbk/1

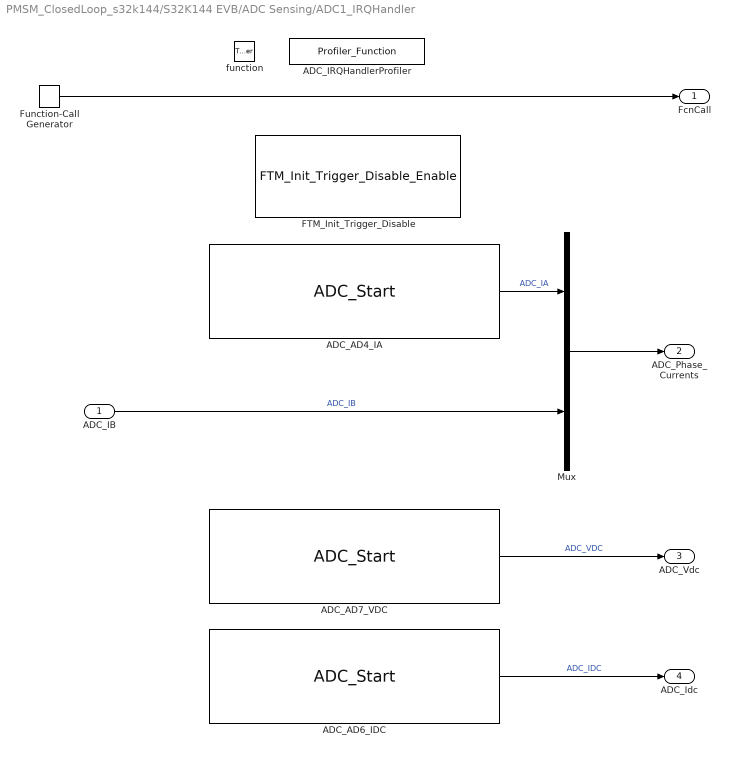
== system PMSM_ClosedLoop_s32k144/S32K144 EVB/ADC Sensing/ADC1_IRQHandler ==
  ADC_IB : Inport
  function : TriggerPort  TriggerType=function-call  VariantControl=(inherit)
  ADC_AD4_IA : mbd_s32k1xx_ec_toolbox/Motor Control Blocks/ADC Blocks/ADC_Start  Priority=2  instance=0  adc_r=A  adc_chan=PTB0: [ADC0_SE4 | ADC Single Ended Input]  aien=off  mcuTargetUpdate=on
  ADC_AD6_IDC : mbd_s32k1xx_ec_toolbox/Motor Control Blocks/ADC Blocks/ADC_Start  Priority=4  instance=1  adc_r=B  adc_chan=PTD4: [ADC1_SE6 | ADC Single Ended Input]  aien=off  mcuTargetUpdate=on
  ADC_AD7_VDC : mbd_s32k1xx_ec_toolbox/Motor Control Blocks/ADC Blocks/ADC_Start  Priority=3  instance=1  adc_r=A  adc_chan=PTB12: [ADC1_SE7 | ADC Single Ended Input]  aien=off  mcuTargetUpdate=on
  ADC_IRQHandlerProfiler : mbd_s32k1xx_ec_toolbox/Utility Blocks/Profiler_Function  profile_indx=0
  FTM_Init_Trigger_Disable : mbd_s32k1xx_ec_toolbox/Motor Control Blocks/FTM Blocks/FTM_Init_Trigger_Disable_Enable  Priority=2  ftmModule=3  action=Disable
  Function-Call Generator : simulink/Ports & Subsystems/Function-Call Generator  sample_time=-1  numberOfIterations=1
  Mux : Mux  Inputs=2
  FcnCall : Outport
  ADC_Phase_Currents : Outport  Port=2
  ADC_Vdc : Outport  Port=3
  ADC_Idc : Outport  Port=4
  wires:
  ADC_AD7_VDC/1 -> ADC_Vdc/1  "ADC_VDC"
  ADC_IB/1 -> Mux/2  "ADC_IB"
  ADC_AD6_IDC/1 -> ADC_Idc/1  "ADC_IDC"
  Function-Call Generator/1 -> FcnCall/1
  Mux/1 -> ADC_Phase_Currents/1
  ADC_AD4_IA/1 -> Mux/1  "ADC_IA"

== system PMSM_ClosedLoop_s32k144/S32K144 EVB/ADC Sensing/PDB1_IRQHandler ==
  function : TriggerPort  TriggerType=function-call  VariantControl=(inherit)
  FTM_Init_Trigger_Enable : mbd_s32k1xx_ec_toolbox/Motor Control Blocks/FTM Blocks/FTM_Init_Trigger_Disable_Enable  ftmModule=3  action=Enable

== system PMSM_ClosedLoop_s32k144/S32K144 EVB/FastLoopControl/Compute_Reference_Voltages ==
  ID_REF : Inport
  IQ_REF : Inport  Port=2
  ID : Inport  Port=3
  IQ : Inport  Port=4
  Current_Controllers_DQ : Subsystem  TreatAsAtomicUnit=on
      settings: RTWSystemCode=Nonreusable function  RTWFcnNameOpts=Use subsystem name
  D-axis Rotor Align : Switch  Criteria=u2 > Threshold
  Execure Align : DataStoreRead  DataStoreName=ExecuteAlign
  Q-axis Rotor Align : Switch  Criteria=u2 > Threshold
  UD_REF : Outport
  UQ_REF : Outport  Port=2
  wires:
  IQ_REF/1 -> Current_Controllers_DQ/4(IQ_REF), Q-axis Rotor Align/1
  D-axis Rotor Align/1 -> UD_REF/1
  Execure Align/1 -> Current_Controllers_DQ/1(Reset), D-axis Rotor Align/2, Q-axis Rotor Align/2
  ID/1 -> Current_Controllers_DQ/3(ID)
  ID_REF/1 -> D-axis Rotor Align/1, Current_Controllers_DQ/2(ID_REF)
  Current_Controllers_DQ/2(UQ_REF) -> Q-axis Rotor Align/3
  IQ/1 -> Current_Controllers_DQ/5(IQ)
  Current_Controllers_DQ/1(UD_REF) -> D-axis Rotor Align/3
  Q-axis Rotor Align/1 -> UQ_REF/1

== system PMSM_ClosedLoop_s32k144/S32K144 EVB/FastLoopControl/PWMCommands ==
  PWM_A : Inport
  PWM_B : Inport  Port=2
  PWM_C : Inport  Port=3
  Control_Logic1 : Subsystem
  FTM_PWM_Config : mbd_s32k1xx_ec_toolbox/Motor Control Blocks/FTM Blocks/FTM_PWM_Config  ftmModule=3  ftmMode=Center-Aligned PWM  ftmSourceClock=80 MHz  swcontrol_enable=off  chan0En=on  chan0Type=Independent  chan2En=on  chan2Type=Independent  chan4En=on  chan4Type=Independent  chan6En=off  chan6Type=Independent  ftmPwmUnits=Hz  outFrequency=20000  ftmPeriod=4000  ftmPrescaler=Divide by 1  deadtimeUnits=Nanoseconds  deadtimeNs=0  deadtimeTicks=0  deadtimePrescaler=Divide by 1  dutyCycleCh0=0  dutyCycleCh1=0  dutyCycleCh2=0  dutyCycleCh3=0  dutyCycleCh4=0  dutyCycleCh5=0  dutyCycleCh6=0.25  dutyCycleCh7=0.25  dutyCycleSim=off  startAfterInit=off  showAdvOpt=on  pinFtmCh0=PTB8: [FTM3_CH0 | FTM Channel]  pinFtmCh1=PTB9: [FTM3_CH1 | FTM Channel]  pinPolCh0=Active Low  pinPolCh1=Active Low  outputComplem0=Main duplicated  outputLevel0=Low  outputLevel1=Low  pinFtmCh2=PTB10: [FTM3_CH2 | FTM Channel]  pinFtmCh3=PTB11: [FTM3_CH3 | FTM Channel]  pinPolCh2=Active Low  pinPolCh3=Active Low  outputComplem2=Main duplicated  outputLevel2=Low  outputLevel3=Low  pinFtmCh4=PTC10: [FTM3_CH4 | FTM Channel]  pinFtmCh5=PTC11: [FTM3_CH5 | FTM Channel]  pinPolCh4=Active Low  pinPolCh5=Active Low  outputComplem4=Main duplicated  outputLevel4=Low  outputLevel5=Low  pinFtmCh6=PTC12: [FTM3_CH6 | FTM Channel]  pinFtmCh7=None  pinPolCh6=Active Low  pinPolCh7=Active Low  outputComplem6=Main duplicated  outputLevel6=Low  outputLevel7=Low  initTrigger=off  chTrigger0=off  chTrigger1=off  chTrigger2=off  chTrigger3=off  chTrigger4=off  chTrigger5=off  chTrigger6=off  chTrigger7=off  mcuTargetUpdate=on  pwmSyncTrg=Software trigger  pwmSyncHwRouting=TRGMUX_FTM7  pwmSyncTrg0=off  pwmSyncTrg1=off  pwmSyncTrg2=off  pwmSyncAutoClear=off  pwmSyncMinLoad=off  pwmSyncMaxLoad=on  pwmSyncInvert=PWM Syncronization  pwmSyncOutControl=PWM Syncronization  pwmSyncOutMask=PWM Syncronization  pwmSyncCounterInitial=PWM Syncronization  pwmSyncPoints=Wait Loading Points  reloadEnable=off  reloadPriority=15  reloadHalfCycle=off  reloadHCR=0  reloadFrequency=0  chnMatch0=off  chnMatch1=off  chnMatch2=off  chnMatch3=off  chnMatch4=off  chnMatch5=off  chnMatch6=off  chnMatch7=off  pwmFaultProtection=off  pwmFaultInterrupt=off  pwmFaultClearing=Fault control disabled  pwmFaultPinState=Safe Value  pwmFaultFilterValue=0  pwmFaultPriority=15  fault_disen_0=off  fault_filter_0=off  fault_polarity_0=Active High  fault_disen_1=off  fault_filter_1=off  fault_polarity_1=Active high  fault_disen_2=off  fault_filter_2=off  fault_polarity_2=Active high  fault_disen_3=off  fault_filter_3=off  fault_polarity_3=Active high  fault_pin_0=None  fault_pin_1=None  fault_pin_2=None  fault_pin_3=None
  wires:
  Control_Logic1/2(PhaseA_LS_out) -> FTM_PWM_Config/2  "PA_LS"
  Control_Logic1/1(PhaseA_HS_out) -> FTM_PWM_Config/1  "PA_HS"
  Control_Logic1/3(PhaseB_HS_out) -> FTM_PWM_Config/3  "PB_HS"
  Control_Logic1/4(PhaseB_LS_out) -> FTM_PWM_Config/4  "PB_LS"
  Control_Logic1/5(PhaseC_HS_out) -> FTM_PWM_Config/5  "PC_HS"
  Control_Logic1/6(PhaseC_LS_out) -> FTM_PWM_Config/6  "PC_LS"
  PWM_A/1 -> Control_Logic1/2(PhaseA_LS), Control_Logic1/1(PhaseA_HS)  "PWM_A"
  PWM_B/1 -> Control_Logic1/4(PhaseB_LS), Control_Logic1/3(PhaseB_HS)  "PWM_B"
  PWM_C/1 -> Control_Logic1/6(PhaseC_LS), Control_Logic1/5(PhaseC_HS)  "PWM_C"

== system PMSM_ClosedLoop_s32k144/S32K144 EVB/FastLoopControl/Rotor_Position ==
  Speed_Reference [rad/s] : Inport
  Align vs. Normal  Operation : Switch  Threshold=1
  ComputeElectricAngle : Subsystem  TreatAsAtomicUnit=on
      settings: RTWSystemCode=Nonreusable function  RTWFcnNameOpts=Use subsystem name
  Execure Align : DataStoreRead  DataStoreName=ExecuteAlign
  ExecureAlign : DataStoreWrite  DataStoreName=THETA
  ModeControl1 : DataStoreRead  DataStoreName=MODE
  Open vs Closed  Loop : Switch  Criteria=u2 > Threshold  Threshold=1
  Standstill : Constant  Value=0  OutDataTypeStr=single  SampleTime=-1
  Sum1 : Sum
  THETA_ESTIMATED_CORRECTED : DataStoreWrite  DataStoreName=THETA_EST_COR
  THETA_EST_CORRECTED : DataStoreRead  DataStoreName=THETA_EST_COR
  THETA_INCREMENT : DataStoreRead  DataStoreName=THETA_INC
  theta : Outport  OutDataTypeStr=single
  wires:
  ModeControl1/1 -> Open vs Closed  Loop/2
  ComputeElectricAngle/1(theta) -> Open vs Closed  Loop/3
  Standstill/1 -> Align vs. Normal  Operation/1
  Sum1/1 -> THETA_ESTIMATED_CORRECTED/1, Open vs Closed  Loop/1
  Execure Align/1 -> Align vs. Normal  Operation/2
  Open vs Closed  Loop/1 -> Align vs. Normal  Operation/3
  THETA_EST_CORRECTED/1 -> Sum1/1
  THETA_INCREMENT/1 -> Sum1/2
  Align vs. Normal  Operation/1 -> theta/1, ExecureAlign/1
  Speed_Reference [rad/s]/1 -> ComputeElectricAngle/1(Speed_Reference [rad/s])

== system PMSM_ClosedLoop_s32k144/S32K144 EVB/IO Controls/Alignment ==
  Action Port : ActionPort
  LED_BLUE : mbd_s32k1xx_ec_toolbox/GPIO Blocks/Digital_Output  gpio_pin=PTD0: [PTD0 | Port D I/O]  init_val=Low  drive_strength=Low
  LED_GREEN : mbd_s32k1xx_ec_toolbox/GPIO Blocks/Digital_Output  gpio_pin=PTD16: [PTD16 | Port D I/O]  init_val=Low  drive_strength=Low
  LED_RED : mbd_s32k1xx_ec_toolbox/GPIO Blocks/Digital_Output  gpio_pin=PTD15: [PTD15 | Port D I/O]  init_val=Low  drive_strength=Low
  OFF : Constant  OutDataTypeStr=boolean
  "OFF " : Constant  OutDataTypeStr=boolean
  Repeating Sequence Stair : simulink/Sources/Repeating Sequence Stair  OutValues=[0 1].'  tsamp=-1  OutMin=[]  OutMax=[]  OutDataTypeStr=fixdt('boolean')  OutputDataTypeScalingMode=Specify via dialog  OutDataType=fixdt('boolean')  ConRadixGroup=Best Precision: Vector-wise  OutScaling=[]
  Zero-Order Hold : ZeroOrderHold  SampleTime=0.1
  wires:
  Zero-Order Hold/1 -> LED_GREEN/1
  Repeating Sequence Stair/1 -> Zero-Order Hold/1
  OFF/1 -> LED_BLUE/1
  "OFF "/1 -> LED_RED/1

== system PMSM_ClosedLoop_s32k144/S32K144 EVB/IO Controls/NormalOp ==
  Action Port : ActionPort
  FAULT : Subsystem  TreatAsAtomicUnit=on
  If : If  IfExpression=(u1 == 0)
  LED_GREEN : mbd_s32k1xx_ec_toolbox/GPIO Blocks/Digital_Output  gpio_pin=PTD16: [PTD16 | Port D I/O]  init_val=Low  drive_strength=Low
  "OFF " : Constant  OutDataTypeStr=boolean
  RUNNING_OK : Subsystem  TreatAsAtomicUnit=on
  SpeedCmd2 : DataStoreRead  DataStoreName=FAULT
  wires:
  If/1 -> RUNNING_OK/Action
  If/2 -> FAULT/Action
  "OFF "/1 -> LED_GREEN/1
  SpeedCmd2/1 -> If/1

== system PMSM_ClosedLoop_s32k144/S32K144 EVB/IO Controls/START ==
  Action Port : ActionPort
  ON : Constant  OutDataTypeStr=boolean
  "SpeedCmd " : DataStoreWrite  DataStoreName=START
  wires:
  ON/1 -> "SpeedCmd "/1

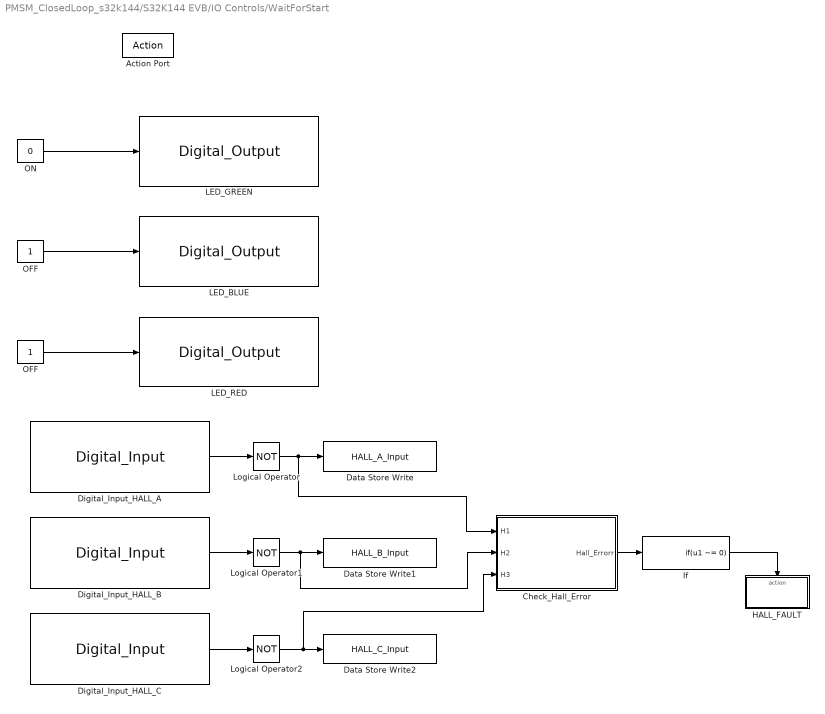
== system PMSM_ClosedLoop_s32k144/S32K144 EVB/IO Controls/WaitForStart ==
  Action Port : ActionPort
  Check_Hall_Error : Subsystem
  Data Store Write : DataStoreWrite  DataStoreName=HALL_A_Input
  Data Store Write1 : DataStoreWrite  DataStoreName=HALL_B_Input
  Data Store Write2 : DataStoreWrite  DataStoreName=HALL_C_Input
  Digital_Input_HALL_A : mbd_s32k1xx_ec_toolbox/GPIO Blocks/Digital_Input  gpio_pin=PTD11: [PTD11 | Port D I/O]  pull_resistor=None  passive_filter=off
  Digital_Input_HALL_B : mbd_s32k1xx_ec_toolbox/GPIO Blocks/Digital_Input  gpio_pin=PTD10: [PTD10 | Port D I/O]  pull_resistor=None  passive_filter=off
  Digital_Input_HALL_C : mbd_s32k1xx_ec_toolbox/GPIO Blocks/Digital_Input  gpio_pin=PTA1: [PTA1 | Port A I/O]  pull_resistor=None  passive_filter=off
  HALL_FAULT : Subsystem  TreatAsAtomicUnit=on
  If : If  IfExpression=u1 ~= 0  ShowElse=off
  LED_BLUE : mbd_s32k1xx_ec_toolbox/GPIO Blocks/Digital_Output  gpio_pin=PTD0: [PTD0 | Port D I/O]  init_val=Low  drive_strength=Low
  LED_GREEN : mbd_s32k1xx_ec_toolbox/GPIO Blocks/Digital_Output  gpio_pin=PTD16: [PTD16 | Port D I/O]  init_val=Low  drive_strength=Low
  LED_RED : mbd_s32k1xx_ec_toolbox/GPIO Blocks/Digital_Output  gpio_pin=PTD15: [PTD15 | Port D I/O]  init_val=Low  drive_strength=Low
  Logical Operator : Logic  Operator=NOT  AllPortsSameDT=off  OutDataTypeStr=boolean
  Logical Operator1 : Logic  Operator=NOT  AllPortsSameDT=off  OutDataTypeStr=boolean
  Logical Operator2 : Logic  Operator=NOT  AllPortsSameDT=off  OutDataTypeStr=boolean
  OFF : Constant  OutDataTypeStr=boolean
  "OFF " : Constant  OutDataTypeStr=boolean
  "ON " : Constant  Value=0  OutDataTypeStr=boolean
  wires:
  "ON "/1 -> LED_GREEN/1
  OFF/1 -> LED_BLUE/1
  "OFF "/1 -> LED_RED/1
  Logical Operator2/1 -> Check_Hall_Error/3(H3), Data Store Write2/1
  Digital_Input_HALL_C/1 -> Logical Operator2/1
  Logical Operator1/1 -> Check_Hall_Error/2(H2), Data Store Write1/1
  Logical Operator/1 -> Check_Hall_Error/1(H1), Data Store Write/1
  Digital_Input_HALL_A/1 -> Logical Operator/1
  Digital_Input_HALL_B/1 -> Logical Operator1/1
  Check_Hall_Error/1(Hall_Errorr) -> If/1
  If/1 -> HALL_FAULT/Action

== system PMSM_ClosedLoop_s32k144/S32K144 EVB/IRQ_Dispatcher/Generate_Triggers ==
  IRQ : TriggerPort  TriggerType=function-call  VariantControl=(inherit)
  Add : Sum  AccumDataTypeStr=uint16  InputSameDT=on
  Function-Call Generator : simulink/Ports & Subsystems/Function-Call Generator  Priority=1  sample_time=-1  numberOfIterations=1
  Keep_Counting : Subsystem  TreatAsAtomicUnit=on
  LoopCounter_read : DataStoreRead  DataStoreName=LoopCounter
  SlowLoop_check : If  IfExpression=u1 >= SPEED_LOOP_CNTR
  Trigger_SlowLoop_Execution : Subsystem  TreatAsAtomicUnit=on
  counter_increment : Constant  OutDataTypeStr=uint16
  FastLoop_Call : Outport
  SlowLoop_Call : Outport  Port=2
  wires:
  Function-Call Generator/1 -> FastLoop_Call/1
  counter_increment/1 -> Add/1
  LoopCounter_read/1 -> Add/2
  SlowLoop_check/1 -> Trigger_SlowLoop_Execution/Action
  Trigger_SlowLoop_Execution/1(Call) -> SlowLoop_Call/1
  Add/1 -> Keep_Counting/1(LoopCounter), SlowLoop_check/1
  SlowLoop_check/2 -> Keep_Counting/Action

== system PMSM_ClosedLoop_s32k144/S32K144 EVB/IRQ_Dispatcher/Trigger_FastLoop_Call ==
  Action Port : ActionPort
  Function-Call Generator : simulink/Ports & Subsystems/Function-Call Generator  sample_time=C_LST  numberOfIterations=1
  Call : Outport
  wires:
  Function-Call Generator/1 -> Call/1

== system PMSM_ClosedLoop_s32k144/S32K144 EVB/Measurements/FaultDetection ==
  Vdc : Inport
  Idc : Inport  Port=2
  ABS : ammclib_bam_s32k14x/MLIB/bam_flt/MLIB_Abs_FLT
  Check_Voltage_Current_Limits : If  NumInputs=2  IfExpression=(u1 < VDC_UNDERVOLTAGE) | (u1 > VDC_OVERVOLTAGE) | (u2 > IDC_OVERCURRENT)  ShowElse=off
  FAILURE : Subsystem  TreatAsAtomicUnit=on
  wires:
  Vdc/1 -> Check_Voltage_Current_Limits/1
  ABS/1 -> Check_Voltage_Current_Limits/2
  Check_Voltage_Current_Limits/1 -> FAILURE/Action
  Idc/1 -> ABS/1

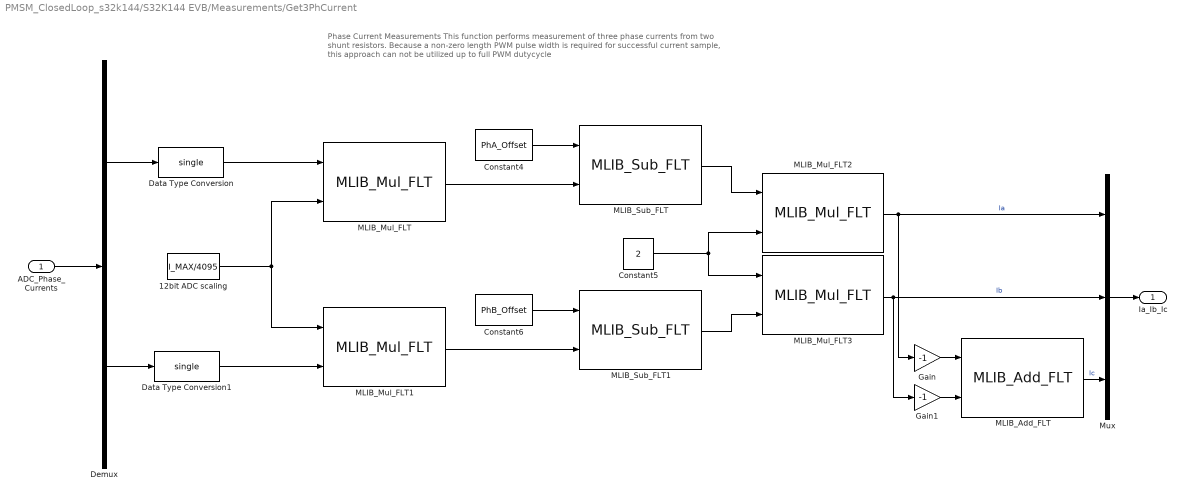
== system PMSM_ClosedLoop_s32k144/S32K144 EVB/Measurements/Get3PhCurrent ==
  note: Phase Current Measurements
      |
      | This function performs measurement of three phase currents from two shunt resistors. Because a non-zero length PWM pulse width is required for successful current sample, this approach can not be utilized up to full PWM dutycycle
  ADC_Phase_Currents : Inport
  12bit ADC scaling : Constant  Value=I_MAX/4095  OutDataTypeStr=single
  Constant4 : Constant  Value=PhA_Offset  OutDataTypeStr=single
  Constant5 : Constant  Value=2  OutDataTypeStr=single
  Constant6 : Constant  Value=PhB_Offset  OutDataTypeStr=single
  Data Type Conversion : DataTypeConversion  OutDataTypeStr=single
  Data Type Conversion1 : DataTypeConversion  OutDataTypeStr=single
  Demux : Demux  Outputs=2
  Gain : Gain  Gain=-1  OutDataTypeStr=single
  Gain1 : Gain  Gain=-1  OutDataTypeStr=single
  MLIB_Add_FLT : ammclib_bam_s32k14x/MLIB/bam_flt/MLIB_Add_FLT
  MLIB_Mul_FLT{,1..3} (4 alike) : ammclib_bam_s32k14x/MLIB/bam_flt/MLIB_Mul_FLT
  MLIB_Sub_FLT : ammclib_bam_s32k14x/MLIB/bam_flt/MLIB_Sub_FLT
  MLIB_Sub_FLT1 : ammclib_bam_s32k14x/MLIB/bam_flt/MLIB_Sub_FLT
  Mux : Mux  Inputs=3
  Ia_Ib_Ic : Outport
  wires:
  Demux/1 -> Data Type Conversion/1
  Mux/1 -> Ia_Ib_Ic/1
  Data Type Conversion/1 -> MLIB_Mul_FLT/1
  MLIB_Mul_FLT/1 -> MLIB_Sub_FLT/2
  MLIB_Mul_FLT1/1 -> MLIB_Sub_FLT1/2
  12bit ADC scaling/1 -> MLIB_Mul_FLT/2, MLIB_Mul_FLT1/1
  Demux/2 -> Data Type Conversion1/1
  MLIB_Mul_FLT2/1 -> Gain/1, Mux/1  "Ia"
  MLIB_Add_FLT/1 -> Mux/3  "Ic"
  Constant4/1 -> MLIB_Sub_FLT/1
  MLIB_Sub_FLT/1 -> MLIB_Mul_FLT2/1
  Constant5/1 -> MLIB_Mul_FLT2/2, MLIB_Mul_FLT3/1
  Constant6/1 -> MLIB_Sub_FLT1/1
  MLIB_Sub_FLT1/1 -> MLIB_Mul_FLT3/2
  MLIB_Mul_FLT3/1 -> Gain1/1, Mux/2  "Ib"
  Gain/1 -> MLIB_Add_FLT/1
  Gain1/1 -> MLIB_Add_FLT/2
  ADC_Phase_Currents/1 -> Demux/1
  Data Type Conversion1/1 -> MLIB_Mul_FLT1/2

== system PMSM_ClosedLoop_s32k144/S32K144 EVB/Measurements/GetIdcCurrent ==
  note: DC-Link Current Measurement
      |
      | This function performs measurement of DC-Bus Current
  ADC_Idc : Inport
  ADC_AD6 offset  and  Logic power supply compensation : Constant  Value=2090  OutDataTypeStr=uint32
  MLIB_Mul_FLT : ammclib_bam_s32k14x/MLIB/bam_flt/MLIB_Mul_FLT
  Sum : Sum  Inputs=+-  OutDataTypeStr=single
  bits2amps : Constant  Value=16.5/2048  OutDataTypeStr=single
  Idc : Outport
  wires:
  bits2amps/1 -> MLIB_Mul_FLT/2
  ADC_Idc/1 -> Sum/1
  ADC_AD6 offset  and  Logic power supply compensation/1 -> Sum/2
  MLIB_Mul_FLT/1 -> Idc/1  "Idc"
  Sum/1 -> MLIB_Mul_FLT/1

== system PMSM_ClosedLoop_s32k144/S32K144 EVB/Measurements/GetVdcVoltage ==
  note: `
  note: DC-Link Voltage Measurement
      |
      | This function performs measurement of DC-Bus Voltage
  ADC_Vdc : Inport
  ADC1_AD7_Offset : Constant  Value=17  OutDataTypeStr=uint32
  Add : Sum  Inputs=-+  AccumDataTypeStr=uint32  OutMin=0  OutMax=4095  OutDataTypeStr=Inherit: Inherit via back propagation  InputSameDT=on
  MLIB_Mul_FLT : ammclib_bam_s32k14x/MLIB/bam_flt/MLIB_Mul_FLT
  bits2volts : Constant  Value=45/4095  OutDataTypeStr=single
  Vdc : Outport
  wires:
  ADC1_AD7_Offset/1 -> Add/1
  ADC_Vdc/1 -> Add/2
  bits2volts/1 -> MLIB_Mul_FLT/2
  Add/1 -> MLIB_Mul_FLT/1
  MLIB_Mul_FLT/1 -> Vdc/1  "Vdc"

== system PMSM_ClosedLoop_s32k144/S32K144 EVB/SlowLoopControl/Alignment_vs_NormalOp_Sequence ==
  Torque_Cmd : Inport
  Flux_Cmd : Inport  Port=2
  D-axis Rotor Align : Switch  Criteria=u2 > Threshold
  Execure Align : DataStoreRead  DataStoreName=ExecuteAlign
  Flux Reference for rotor alignment : Constant  Value=0.1  OutDataTypeStr=single  SampleTime=-1
  Q-axis Rotor Align : Switch  Criteria=u2 > Threshold
  Torque Reference  for Alignment : Constant  Value=0  OutDataTypeStr=single  SampleTime=-1
  Torque_Ref : Outport
  Flux_Ref : Outport  Port=2
  wires:
  Execure Align/1 -> Q-axis Rotor Align/2, D-axis Rotor Align/2
  Flux_Cmd/1 -> D-axis Rotor Align/3
  Torque Reference  for Alignment/1 -> Q-axis Rotor Align/1
  Q-axis Rotor Align/1 -> Torque_Ref/1
  Torque_Cmd/1 -> Q-axis Rotor Align/3
  Flux Reference for rotor alignment/1 -> D-axis Rotor Align/1
  D-axis Rotor Align/1 -> Flux_Ref/1
